simulink model "Inverter"  (R2017b)
settings: Solver=VariableStepAuto  StartTime=0.0  StopTime=1  MaxStep=1e-4  RelTol=1e-3
libraries: powerlib x11
settings Model: Creator=DELL  LastModifiedBy=DELL

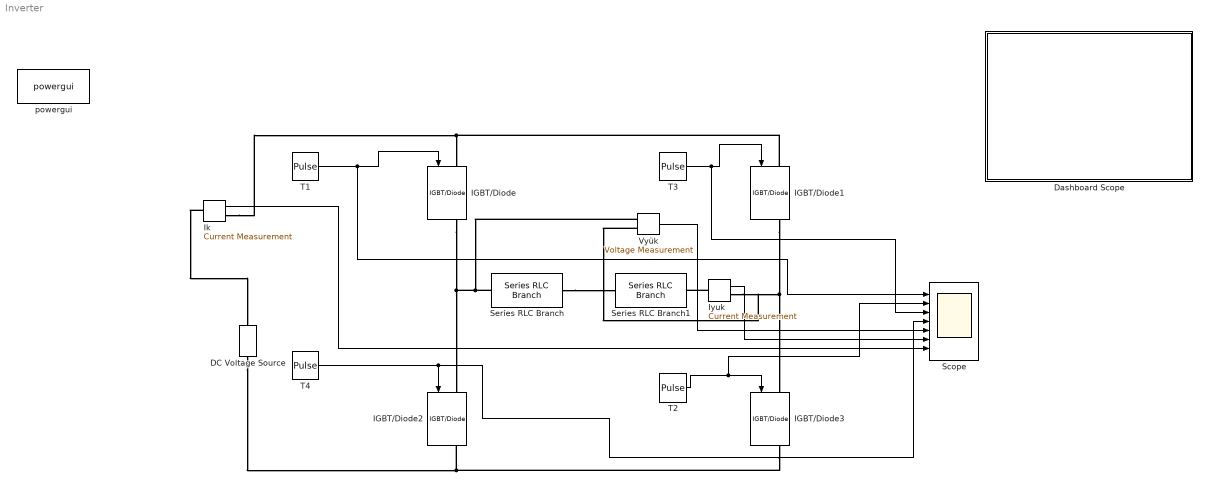
== system Inverter ==
  DC Voltage Source : powerlib/Electrical Sources/DC Voltage Source  Amplitude=120  Measurements=None
  Dashboard Scope : Subsystem  DialogController=hmiCreateDDGDialog  IsWebBlock=on  mask(MWDashboardBlock){webBlockId=7297c926-ad48-4129-872b-47a6d69f0cdb, webBlockType=sdiscope, ShowInitialText=on, HMISrcModelName=Evirici}
      mask prompts: webBlockId "WebBlock Id"; webBlockType "WebBlock Type"; HMISrcModelName "Source Model"
      mask help: SimulinkHMI:dialogs:HMIScopeDialogDesc
      mask Help: helpview([docroot '/mapfiles/simulink.map'], 'hmi_scope')
      mask Display:
      | if strcmp(get_param(bdroot(gcb),'BlockDiagramType'), 'library')
      |     image([(matlabroot) '/toolbox/simulink/hmi/icons/DashboardScope.png']);
      | end
  IGBT/Diode{,1..3} (4 alike) : powerlib/Power Electronics/IGBT//Diode  Ron=1e-3  Rs=1e5  Cs=inf  Measurements=on
  Ik : powerlib/Measurements/Current Measurement  PhasorSimulation=off  OutputType=Complex  PSBequivalent=0
  Iyuk : powerlib/Measurements/Current Measurement  PhasorSimulation=off  OutputType=Complex  PSBequivalent=0
  Scope : Scope  NumInputPorts=7
  Series RLC Branch : powerlib/Elements/Series RLC Branch  LConnTagsString=__new0  RConnTagsString=__new0  BranchType=R  Resistance=2  Inductance=1e-3  SetiL0=off  InitialCurrent=0  Capacitance=1e-6  Setx0=off  InitialVoltage=0  Measurements=None
  Series RLC Branch1 : powerlib/Elements/Series RLC Branch  LConnTagsString=__new0  RConnTagsString=__new0  BranchType=L  Resistance=1  Inductance=20e-3  SetiL0=off  InitialCurrent=0  Capacitance=1e-6  Setx0=off  InitialVoltage=0  Measurements=None
  T1 : DiscretePulseGenerator  PulseType=Time based  Period=0.01666  PulseWidth=50  PhaseDelay=0.01666*151.2/360
  T2 : DiscretePulseGenerator  PulseType=Time based  Period=0.01666  PulseWidth=50  PhaseDelay=0.01666*302.4/360
  T3 : DiscretePulseGenerator  PulseType=Time based  Period=0.01666  PulseWidth=50  PhaseDelay=0.01666*122.4/360
  T4 : DiscretePulseGenerator  PulseType=Time based  Period=0.01666  PulseWidth=50  PhaseDelay=0.01666*331.2/360
  Vyük : powerlib/Measurements/Voltage Measurement  PhasorSimulation=off  OutputType=Complex  PSBequivalent=0
  powergui : powerlib/powergui  Priority=1  SimulationMode=Continuous  SampleTime=50e-6  frequency=60  Iterations=50  frequencyindice=0  Pbase=100e6  ErrMax=1e-4  UnitsV=kV  UnitsW=MW  buscounter=0  FunctionMessages=off  echomessages=off  EnableUseOfTLC=off  CurrentSourceSwitches=off  DisableSnubberDevices=off  DisableRonSwitches=off  DisableVfSwitches=off  DisplayEquations=off  SolverType=Tustin/Backward Euler (TBE)  Interpol=off  ExternalGateDelay=off  methode=off  Ts=100  x0status=blocks  SPID=on  SwTol=0  HookPort=off  RestoreLinks=warning  ResistiveCurrentMeasurement=off  Frange=[0:2:500]  Ylog=off  Xlog=on  ShowGrid=off  save=off  variable=ZData  structure=0  ZoomFFT=off  StartTime=0.0  cycles=1  DisplayStyle=1  fundamental=60  FreqAxis=off  MaxFrequency=1000  frequencyindicesteady=1  RmsSteady=1  display=off
  wires:
  T3/1 -> Scope/3, IGBT/Diode1/1
  T1/1 -> Scope/1, IGBT/Diode/1
  T4/1 -> Scope/4, IGBT/Diode2/1
  T2/1 -> Scope/2, IGBT/Diode3/1
  Vyük/1 -> Scope/5
  Iyuk/1 -> Scope/6
  Ik/1 -> Scope/7
  connections:
  Series RLC Branch/RConn1 -- Series RLC Branch1/LConn1
  Series RLC Branch/LConn1 -- Vyük/LConn1 -- IGBT/Diode2/LConn1 -- IGBT/Diode/RConn1
  IGBT/Diode1/RConn1 -- Vyük/LConn2 -- Iyuk/RConn1 -- IGBT/Diode3/LConn1
  IGBT/Diode1/LConn1 -- IGBT/Diode/LConn1 -- Ik/RConn1
  Iyuk/LConn1 -- Series RLC Branch1/RConn1
  Ik/LConn1 -- DC Voltage Source/RConn1
  IGBT/Diode3/RConn1 -- DC Voltage Source/LConn1 -- IGBT/Diode2/RConn1

== system Inverter/Dashboard Scope ==
